simulink model "MinSegShield_Demo_M1V4"  (R2013a)
settings: Solver=FixedStepDiscrete  SolverMode=SingleTasking  StartTime=0.0  StopTime=inf  FixedStep=.1  RelTol=1e-3
libraries: arduinolib x4, MinSegLibrary_M1V4 x2
settings Model: SimulationMode=external  ExtModeTrigDuration=2  Creator=Alec  LastModifiedBy=hurstj
settings OptimizationCC: ExpressionDepthLimit=2147483647  OptimizeModelRefInitCode=on  LifeSpan=1
settings DebuggingCC: SolverPrmCheckMsg=none  StrictBusMsg=Warning
settings HardwareCC: ProdBitPerInt=16  ProdBitPerPointer=8  ProdIntDivRoundTo=Zero  ProdEndianess=LittleEndian  ProdWordSize=8  ProdHWDeviceType=Atmel->AVR
settings RTWCC: SystemTargetFile=realtime.tlc  GenerateMakefile=off  TemplateMakefile=realtime.tmf  Description=Real-Time Toolbox  RTWVerbose=off  ProcessScript=realtime_make_rtw_hook
settings CodeAppCC: CustomSymbolStrType=$N$R$M  InternalIdentifier=Classic
settings STFCustomTargetCC: TargetLibSuffix=.a  GenerateSampleERTMain=on  ERTCustomFileBanners=on  SupportNonInlinedSFcns=off  SupportVariableSizeSignals=on  MATLABClassNameForMDSCustomization=Simulink.SoftwareTarget.ERTCustomization  SystemTargetFile=realtime.tlc
settings ERTTargetCC: ParMdlRefBuildCompliant=off  CompOptLevelCompliant=off  ConcurrentExecutionCompliant=off  CombineOutputUpdateFcns=off  ERTFirstTimeCompliant=off  SupportContinuousTime=on  SupportVariableSizeSignals=on  ModelStepFunctionPrototypeControlCompliant=off  CPPClassGenCompliant=off  ExtMode=on  ExtModeTransport=3  ExtModeMexFile=ext_serial_win32_comm  ExtModeMexArgs=0 72 115200  ERTSrcFileBannerTemplate=realtime_code_template.cgt  ERTHdrFileBannerTemplate=realtime_code_template.cgt  ERTDataSrcFileTemplate=realtime_code_template.cgt  ERTDataHdrFileTemplate=realtime_code_template.cgt  ERTCustomFileTemplate=realtime_file_process.tlc

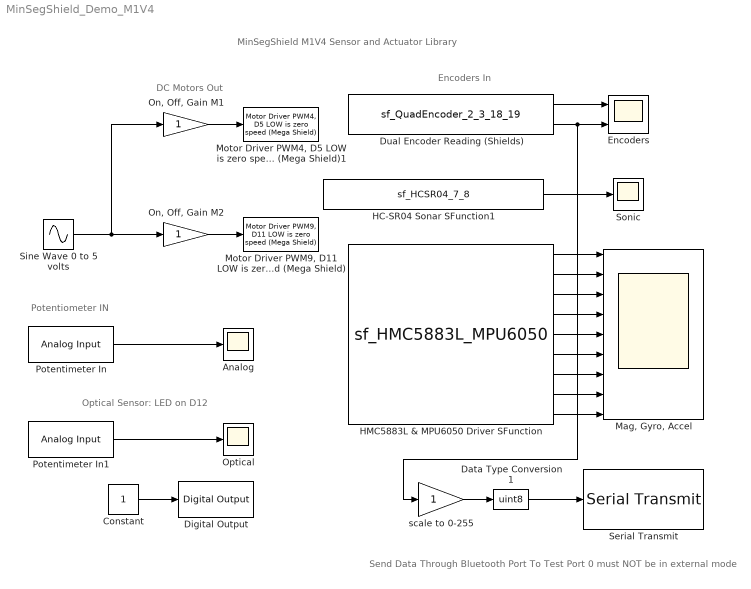
== system MinSegShield_Demo_M1V4 ==
  note: Send Data Through Bluetooth Port
      | To Test Port 0 must NOT be in external mode
  note: Potentiometer IN
  note: DC Motors Out
  note: Encoders In
  note: Optical Sensor: LED on D12
  note: MinSegShield M1V4 Sensor and Actuator Library
  Analog : Scope
      settings: TimeRange=30  YMin=200  YMax=1100  SaveName=ScopeData6
  Constant : Constant
  Data Type Conversion1 : DataTypeConversion  OutDataTypeStr=uint8
  Digital Output : arduinolib/Digital Output  pinNumber=12
  Dual Encoder Reading (Shields) : S-Function  InitFcn=try, set_param(gcb,'FunctionName','sf_QuadEncoder_2_3_18_19'), end  FunctionName=sf_QuadEncoder_2_3_18_19  Parameters=uint8([0 1]),uint8([2 18]),uint8([3 19])  SFunctionModules=sf_QuadEncoder_2_3_18_19_wrapper  EnableBusSupport=off  mask(S-Function Builder){}
      mask init:
      | val = [[.9  0.75 0.75 1 1 .9 .9 1]',[1 1 0.75 0.75 .9 .9 1 .9]'];try , sys = get_param(gcb,'SfunBuilderFcnName');if isempty(sys), sys = get_param(gcb,'FunctionName'); end,catch, sys = get_param(gcb,'FunctionName'); end
      settings: CopyFcn=set_param(gcbh,'LinkStatus','none')  PreSaveFcn=try, set_param(gcb,'FunctionName','sf_QuadEncoder_2_3_18_19'), end  OpenFcn=sfunctionwizard(gcbh)
      mask Display: plot(val(:,1),val(:,2)),disp(sys), port_label('output',1,'pos1'), port_label('output',2,'pos2')
  Encoders : Scope  NumInputPorts=2
      settings: TimeRange=10  YMin=-700~-1  YMax=0~1
  HC-SR04 Sonar SFunction1 : S-Function  InitFcn=try, set_param(gcb,'FunctionName','sf_HCSR04_7_8'), end  FunctionName=sf_HCSR04_7_8  SFunctionModules=sf_HCSR04_7_8_wrapper  EnableBusSupport=off  mask(S-Function Builder){}
      mask help: Simulink:masks:SFunctionBuilder_MD
      mask init: same as MinSegShield_Demo_M1V4/Dual Encoder Reading (Shields)
      settings: CopyFcn=set_param(gcbh,'LinkStatus','none')  PreSaveFcn=try, set_param(gcb,'FunctionName','sf_HCSR04_7_8'), end  OpenFcn=sfunctionwizard(gcbh)
      mask Display:
      | plot(val(:,1),val(:,2))
      | disp(sys)
      | port_label('output',1,'distance_cm')
  HMC5883L & MPU6050 Driver SFunction : S-Function  InitFcn=try, set_param(gcb,'FunctionName','sf_HMC5883L_MPU6050'), end  FunctionName=sf_HMC5883L_MPU6050  SFunctionModules=sf_HMC5883L_MPU6050_wrapper  EnableBusSupport=off  mask(S-Function Builder){}
      mask help: Simulink:masks:SFunctionBuilder_MD
      mask init: same as MinSegShield_Demo_M1V4/Dual Encoder Reading (Shields)
      settings: CopyFcn=set_param(gcbh,'LinkStatus','none')  PreSaveFcn=try, set_param(gcb,'FunctionName','sf_HMC5883L_MPU6050'), end  OpenFcn=sfunctionwizard(gcbh)
      mask Display:
      | plot(val(:,1),val(:,2))
      | disp(sys)
      | port_label('output',1,'x_mag')
      | port_label('output',2,'y_mag')
      | port_label('output',3,'z_mag')
      | port_label('output',4,'x_vel')
      | port_label('output',5,'y_vel')
      | port_label('output',6,'z_vel')
      | port_label('output',7,'x_acc')
      | port_label('output',8,'y_acc')
      | port_label('output',9,'z_acc')
  "Mag, Gyro, Accel" : Scope  NumInputPorts=9
      settings: TimeRange=10  YMin=-1~-1~-1~-20000~-15000~-30000~-4000~-8000~12000  YMax=1~1~1~15000~15000~30000~8000~2000~18000
  "Motor Driver PWM4, D5 LOW is zero speed (Mega Shield)1" : MinSegLibrary_M1V4/Motor Driver PWM4, D5 LOW is zero speed (Mega Shield)  Vsupply=4.5  PWMoffset=0
  "Motor Driver PWM9, D11 LOW is zero speed (Mega Shield)" : MinSegLibrary_M1V4/Motor Driver PWM9, D11 LOW is zero speed (Mega Shield)  Vsupply=4.5  PWMoffset=0
  "On, Off, Gain M1" : Gain  OutDataTypeStr=int16
  "On, Off, Gain M2" : Gain  OutDataTypeStr=int16
  Optical : Scope
      settings: TimeRange=30  YMin=200  YMax=1100  SaveName=ScopeData3
  Potentimeter In : arduinolib/Analog Input  pinNumber=0  sampleTime=-1
  Potentimeter In1 : arduinolib/Analog Input  pinNumber=1  sampleTime=-1
  Serial Transmit : arduinolib/Serial Transmit  portNumber=2
  Sine Wave 0 to 5 volts : Sin  SineType=Sample based  Amplitude=5  Frequency=50*2*pi  Samples=30  SampleTime=.1
  Sonic : Scope
      settings: TimeRange=30  YMin=0  YMax=175  SaveName=ScopeData2
  scale to 0-255 : Gain  OutDataTypeStr=int16
  wires:
  "On, Off, Gain M1"/1 -> "Motor Driver PWM4, D5 LOW is zero speed (Mega Shield)1"/1
  Sine Wave 0 to 5 volts/1 -> "On, Off, Gain M2"/1, "On, Off, Gain M1"/1
  "On, Off, Gain M2"/1 -> "Motor Driver PWM9, D11 LOW is zero speed (Mega Shield)"/1
  Dual Encoder Reading (Shields)/1 -> Encoders/1
  Dual Encoder Reading (Shields)/2 -> scale to 0-255/1, Encoders/2
  HMC5883L & MPU6050 Driver SFunction/1 -> "Mag, Gyro, Accel"/1
  HMC5883L & MPU6050 Driver SFunction/2 -> "Mag, Gyro, Accel"/2
  HMC5883L & MPU6050 Driver SFunction/3 -> "Mag, Gyro, Accel"/3
  HMC5883L & MPU6050 Driver SFunction/4 -> "Mag, Gyro, Accel"/4
  HMC5883L & MPU6050 Driver SFunction/5 -> "Mag, Gyro, Accel"/5
  HMC5883L & MPU6050 Driver SFunction/6 -> "Mag, Gyro, Accel"/6
  HMC5883L & MPU6050 Driver SFunction/7 -> "Mag, Gyro, Accel"/7
  HMC5883L & MPU6050 Driver SFunction/8 -> "Mag, Gyro, Accel"/8
  HMC5883L & MPU6050 Driver SFunction/9 -> "Mag, Gyro, Accel"/9
  scale to 0-255/1 -> Data Type Conversion1/1
  Data Type Conversion1/1 -> Serial Transmit/1
  Potentimeter In/1 -> Analog/1
  HC-SR04 Sonar SFunction1/1 -> Sonic/1
  Potentimeter In1/1 -> Optical/1
  Constant/1 -> Digital Output/1
